simulink model "SingleLinkManipulator"  (R2021a)
settings: Solver=ode14x  StartTime=0.0  StopTime=10.0  RelTol=1e-3
model workspace (MAT data in the model file):
  g = 9.8
  l = 1
  mass = 3
  nu = 6
values from neighbouring files (symbols this model uses):
  F_input = reshape(F{1, 1}, [], 1)    [simulink_state_update_fn.m]
  X1_0 = reshape(X{1, 1}, [], 1)    [simulink_state_update_fn.m]
  X2_0 = reshape(X{1, 2}, [], 1)    [simulink_state_update_fn.m]
settings Model: Creator=adekoyoa  LastModifiedBy=adekoyoa

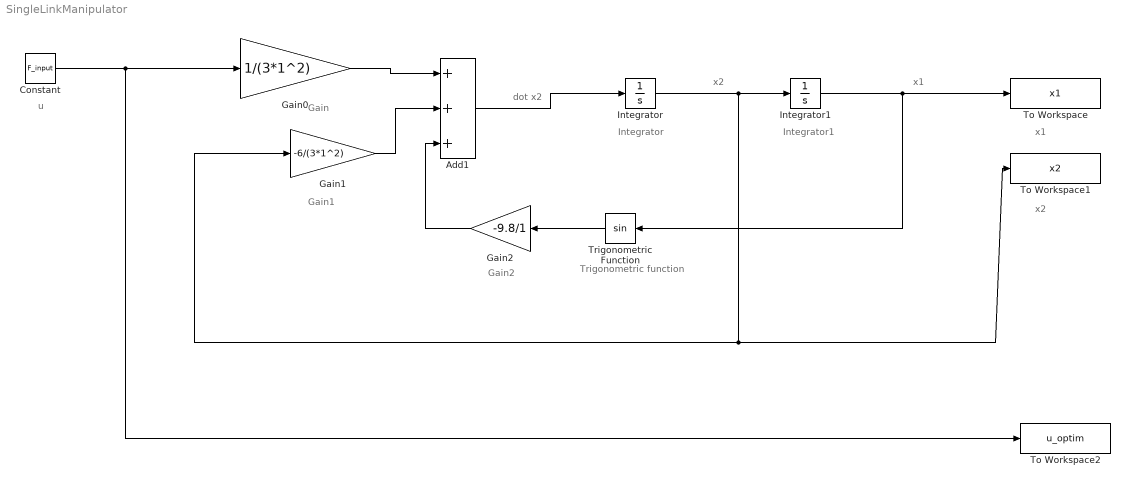
== system SingleLinkManipulator ==
  note: u
  note: Gain2
  note: Trigonometric function
  note: Gain1
  note: Gain
  note: Integrator
  note: Integrator1
  note: x1
  note: x2
  note: dot x2
  note: x2
  note: x1
  Add1 : Sum  Inputs=+++
  Constant : Constant  Value=F_input
  Gain0 : Gain  Gain=1/(3*1^2)
  Gain1 : Gain  Gain=-6/(3*1^2)
  Gain2 : Gain  Gain=-9.8/1
  Integrator : Integrator  InitialCondition=X2_0
  Integrator1 : Integrator  InitialCondition=X1_0
  To Workspace : ToWorkspace  VariableName=x1  SampleTime=-1
  To Workspace1 : ToWorkspace  VariableName=x2  SampleTime=-1
  To Workspace2 : ToWorkspace  VariableName=u_optim  SampleTime=-1
  Trigonometric Function : Trigonometry
  wires:
  Constant/1 -> To Workspace2/1, Gain0/1
  Gain0/1 -> Add1/1
  Gain1/1 -> Add1/2
  Gain2/1 -> Add1/3
  Add1/1 -> Integrator/1
  Integrator/1 -> Gain1/1, To Workspace1/1, Integrator1/1
  Integrator1/1 -> To Workspace/1, Trigonometric Function/1
  Trigonometric Function/1 -> Gain2/1
